simulink model "GridN4"  (R2021a)
settings: Solver=FixedStepAuto  StartTime=0.0  StopTime=0.2  FixedStep=0.2  RelTol=1e-3
libraries: spsDistributedParametersLineLib x13, spsThreePhaseSeriesRLCLoadLib x6, spsThreePhaseVIMeasurementLib x2, spsGroundLib x1, spsThreePhaseSourceLib x1, spsSeriesRLCBranchLib x1, spspowerguiLib x1
settings Model: Creator=miair  LastModifiedBy=Admin
settings SolverCC: AlgebraicLoopSolver=TrustRegion
settings DataIOCC: ReturnWorkspaceOutputs=off
settings DebuggingCC: SFMachineParentedDataDiag=warning  ArithmeticOperatorsInVariantConditions=warning
settings SFSimCC: SimUseLocalCustomCode=off  CustomCodeUndefinedFunction=UseInterfaceOnly
settings RTWCC: RTWUseLocalCustomCode=off
settings CodeAppCC: StateflowObjectComments=on
settings SimscapeCC: SimscapeNormalizeSystem=off

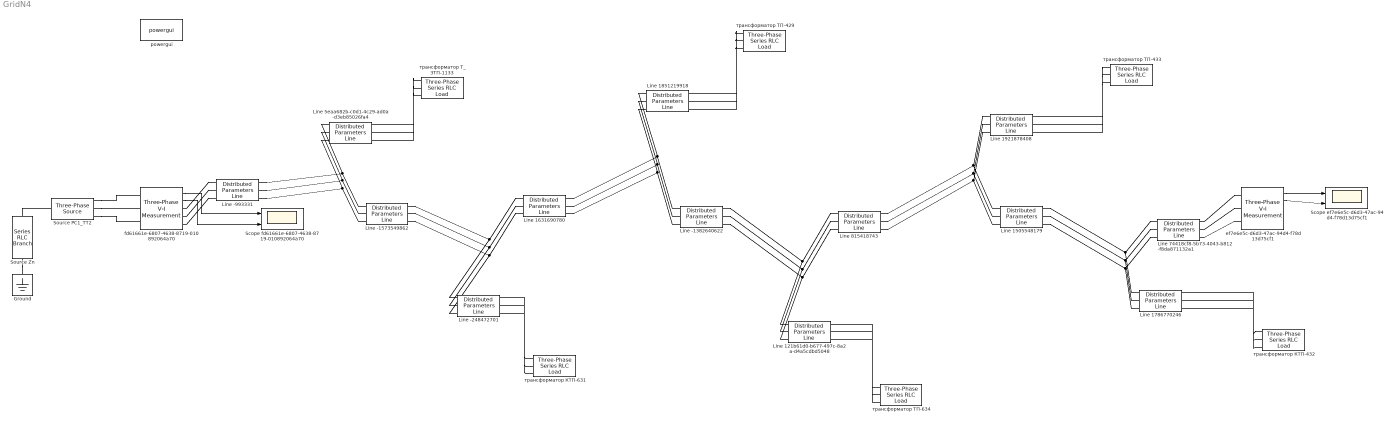
== system GridN4 ==
  Ground : spsGroundLib/Ground  LConnTagsString=a
  Line -1382640622 : spsDistributedParametersLineLib/Distributed Parameters Line  Description=|  Phases=3  Length=1.4772  Frequency=50  Resistance=[0.646656091154803 0.0486237908083191 0.0486712220507153;0.0486237908083191 0.646561225344642 0.0486237934466192;0.0486712220507153 0.0486237934466192 0.646656091154803]  Inductance=[0.00282448912315926 0.00133270803418135 0.00132951476746136;0.00133270803418135 0.00282479813276775 0.00133799988507366;0.00132951476746136 0.00133799988507366 0.00282448912315926]  Capacitance=[7.89543174552926e-09 -1.85986777702161e-09 -1.7901190036642e-09;-1.85986777702161e-09 7.82540023894543e-09 -1.8957321828871e-09;-1.7901190036642e-09 -1.8957321828871e-09 7.91264394645417e-09]  x1=[85.8857792377858 6510.87905206758 6510.37512083704;314.159265358979 314.159265358979 314.159265358979;0.297795361599447 -0.904054654199639 -2.47497799182329]  x2=[85.9647541006012 6498.88512116897 6498.39920566151;314.159265358979 314.159265358979 314.159265358979;0.29836012891069 -0.904731827544364 -2.47564826583381]  x3=[0.104217124772641 6.72029956175141 6.82412580592181;314.159265358979 314.159265358979 314.159265358979;0.111414320617144 -0.3562443922381 -1.93698471339142]  x4=[0.0514466308166242 27.5442395111353 27.6704588799536;314.159265358979 314.159265358979 314.159265358979;0.679987114816006 -1.03294818731528 -2.60316864161815]  x5=7.07796349106919e-06  V1=ones(3,3)  V2=ones(3,3)  I1=ones(3,3)  I2=ones(3,3)  nHarmo=1  Measurements=None  Decoupling=off  VsMag0=0  VrMag0=0  VsAngle0=0  VrAngle0=0  IsMag0=0  IrMag0=0  IsAngle0=0  IrAngle0=0
      | Line connected to devices: [Опора-4/1_Л-8-10кВ_Воробьево
      | Опора-2/44_Л-8-10кВ_Воробьево, Опора-2/67_Л-8-10кВ_Воробьево]
      settings: SourceProductBaseCode=PS
  Line -1573549862 : spsDistributedParametersLineLib/Distributed Parameters Line  Description=|  Phases=3  Length=0.98898  Frequency=50  Resistance=[0.646656091154803 0.0486237908083191 0.0486712220507153;0.0486237908083191 0.646561225344642 0.0486237934466192;0.0486712220507153 0.0486237934466192 0.646656091154803]  Inductance=[0.00282448912315926 0.00133270803418135 0.00132951476746136;0.00133270803418135 0.00282479813276775 0.00133799988507366;0.00132951476746136 0.00133799988507366 0.00282448912315926]  Capacitance=[7.89543174552926e-09 -1.85986777702161e-09 -1.7901190036642e-09;-1.85986777702161e-09 7.82540023894543e-09 -1.8957321828871e-09;-1.7901190036642e-09 -1.8957321828871e-09 7.91264394645417e-09]  x1=[85.6677259618718 6543.90351776437 6543.34962523968;314.159265358979 314.159265358979 314.159265358979;0.296971250306257 -0.901609957237111 -2.47255157035452]  x2=[85.7598900271541 6529.94544416512 6529.41271684245;314.159265358979 314.159265358979 314.159265358979;0.297631180119223 -0.902394975430767 -2.473328653112]  x3=[0.127076602259962 6.46782645683811 6.42234305042791;314.159265358979 314.159265358979 314.159265358979;0.0294613778206171 1.00930239141356 -0.579244928461238]  x4=[0.0432092930617411 35.9185691148936 36.0457502607365;314.159265358979 314.159265358979 314.159265358979;1.18518823340833 -1.07311367571862 -2.64327629161882]  x5=4.73867068331817e-06  V1=ones(3,3)  V2=ones(3,3)  I1=ones(3,3)  I2=ones(3,3)  nHarmo=1  Measurements=None  Decoupling=off  VsMag0=0  VrMag0=0  VsAngle0=0  VrAngle0=0  IsMag0=0  IrMag0=0  IsAngle0=0  IrAngle0=0
      | Line connected to devices: [СШ ЗТП-1133, Опора-3/1_Л-8-10кВ_Воробьево
      | Опора-2/16_Л-8-10кВ_Воробьево]
      settings: SourceProductBaseCode=PS
  Line -248472701 : spsDistributedParametersLineLib/Distributed Parameters Line  Description=|  Phases=3  Length=0.18015  Frequency=50  Resistance=[0.646656091154803 0.0486237908083191 0.0486712220507153;0.0486237908083191 0.646561225344642 0.0486237934466192;0.0486712220507153 0.0486237934466192 0.646656091154803]  Inductance=[0.00282448912315926 0.00133270803418135 0.00132951476746136;0.00133270803418135 0.00282479813276775 0.00133799988507366;0.00132951476746136 0.00133799988507366 0.00282448912315926]  Capacitance=[7.89543174552926e-09 -1.85986777702161e-09 -1.7901190036642e-09;-1.85986777702161e-09 7.82540023894543e-09 -1.8957321828871e-09;-1.7901190036642e-09 -1.8957321828871e-09 7.91264394645417e-09]  x1=[85.7598900271543 6529.94544416512 6529.41271684245;314.159265358979 314.159265358979 314.159265358979;0.298848700228514 -0.901427735668235 -2.4723604926057]  x2=[85.763454791984 6529.39738401349 6528.86547736649;314.159265358979 314.159265358979 314.159265358979;0.298874766091125 -0.901458260199312 -2.47239070103001]  x3=[0.0855260327133963 12.6404163140629 12.764989480605;314.159265358979 314.159265358979 314.159265358979;0.215972029306597 -0.796300987449647 -2.3683442154795]  x4=[0.0651073125741442 20.6999331634113 20.8266702112825;314.159265358979 314.159265358979 314.159265358979;0.407523776195381 -0.965746971947712 -2.53623983661103]  x5=8.63183809176898e-07  V1=ones(3,3)  V2=ones(3,3)  I1=ones(3,3)  I2=ones(3,3)  nHarmo=1  Measurements=None  Decoupling=off  VsMag0=0  VrMag0=0  VsAngle0=0  VrAngle0=0  IsMag0=0  IrMag0=0  IsAngle0=0  IrAngle0=0
      | Line connected to devices: [Опора-3/1_Л-8-10кВ_Воробьево
      | Опора-2/16_Л-8-10кВ_Воробьево, трансформатор КТП-631]
      settings: SourceProductBaseCode=PS
  Line -993331 : spsDistributedParametersLineLib/Distributed Parameters Line  Description=Line connected to devices: [ВВ Ячейка_Л-8-10кВ_Воробьево, СШ ЗТП-1133]  Phases=3  Length=0.892  Frequency=50  Resistance=[0.646656091154803 0.0486237908083191 0.0486712220507153;0.0486237908083191 0.646561225344642 0.0486237934466192;0.0486712220507153 0.0486237934466192 0.646656091154803]  Inductance=[0.00282448912315926 0.00133270803418135 0.00132951476746136;0.00133270803418135 0.00282479813276775 0.00133799988507366;0.00132951476746136 0.00133799988507366 0.00282448912315926]  Capacitance=[7.89543174552926e-09 -1.85986777702161e-09 -1.7901190036642e-09;-1.85986777702161e-09 7.82540023894543e-09 -1.8957321828871e-09;-1.7901190036642e-09 -1.8957321828871e-09 7.91264394645417e-09]  x1=[85.5017510654121 6569.24560507323 6568.65333179846;314.159265358979 314.159265358979 314.159265358979;0.295910641359064 -0.900082774080867 -2.47103868556443]  x2=[85.667725961872 6543.90351776437 6543.34962523968;314.159265358979 314.159265358979 314.159265358979;0.297117232898643 -0.901493983655308 -2.47243548637407]  x3=[0.183284202527258 24.4320765018378 24.3241695261716;314.159265358979 314.159265358979 314.159265358979;-0.0762727108476125 1.71053738269408 0.137523096986334]  x4=[0.0699142754394648 55.8037793342115 55.9323018365664;314.159265358979 314.159265358979 314.159265358979;2.17390443481334 -1.12439915077923 -2.69462173279304]  x5=4.27399365964914e-06  V1=ones(3,3)  V2=ones(3,3)  I1=ones(3,3)  I2=ones(3,3)  nHarmo=1  Measurements=None  Decoupling=off  VsMag0=0  VrMag0=0  VsAngle0=0  VrAngle0=0  IsMag0=0  IrMag0=0  IsAngle0=0  IrAngle0=0
      settings: SourceProductBaseCode=PS
  Line 121b61d0-b677-497c-8a2a-d4a5cdbd5048 : spsDistributedParametersLineLib/Distributed Parameters Line  Description=Line connected to devices: [Опора-2/67_Л-8-10кВ_Воробьево, трансформатор ТП-634]  Phases=3  Length=0.01635  Frequency=50  Resistance=[0.646656091154803 0.0486237908083191 0.0486712220507153;0.0486237908083191 0.646561225344642 0.0486237934466192;0.0486712220507153 0.0486237934466192 0.646656091154803]  Inductance=[0.00282448912315926 0.00133270803418135 0.00132951476746136;0.00133270803418135 0.00282479813276775 0.00133799988507366;0.00132951476746136 0.00133799988507366 0.00282448912315926]  Capacitance=[7.89543174552926e-09 -1.85986777702161e-09 -1.7901190036642e-09;-1.85986777702161e-09 7.82540023894543e-09 -1.8957321828871e-09;-1.7901190036642e-09 -1.8957321828871e-09 7.91264394645417e-09]  x1=[85.9647541006012 6498.88512116897 6498.39920566151;314.159265358979 314.159265358979 314.159265358979;0.300559125302584 -0.902984869336713 -2.47389964464565]  x2=[85.9650422946656 6498.84085463915 6498.3550050936;314.159265358979 314.159265358979 314.159265358979;0.300561215685984 -0.902987343814113 -2.47390209345756]  x3=[0.0845031718933416 12.9941072057686 13.1185063261115;314.159265358979 314.159265358979 314.159265358979;0.225790596837781 -0.81181384254389 -2.38366283032811]  x4=[0.0663567082392332 20.1717718047634 20.2980663663425;314.159265358979 314.159265358979 314.159265358979;0.395804226320378 -0.961685203465561 -2.53219107175892]  x5=7.83405788511923e-08  V1=ones(3,3)  V2=ones(3,3)  I1=ones(3,3)  I2=ones(3,3)  nHarmo=1  Measurements=None  Decoupling=off  VsMag0=0  VrMag0=0  VsAngle0=0  VrAngle0=0  IsMag0=0  IrMag0=0  IsAngle0=0  IrAngle0=0
      settings: SourceProductBaseCode=PS
  Line 1505548179 : spsDistributedParametersLineLib/Distributed Parameters Line  Description=|  Phases=3  Length=0.64126  Frequency=50  Resistance=[0.646656091154803 0.0486237908083191 0.0486712220507153;0.0486237908083191 0.646561225344642 0.0486237934466192;0.0486712220507153 0.0486237934466192 0.646656091154803]  Inductance=[0.00282448912315926 0.00133270803418135 0.00132951476746136;0.00133270803418135 0.00282479813276775 0.00133799988507366;0.00132951476746136 0.00133799988507366 0.00282448912315926]  Capacitance=[7.89543174552926e-09 -1.85986777702161e-09 -1.7901190036642e-09;-1.85986777702161e-09 7.82540023894543e-09 -1.8957321828871e-09;-1.7901190036642e-09 -1.8957321828871e-09 7.91264394645417e-09]  x1=[85.9782141140988 6496.83974420136 6496.35689426354;314.159265358979 314.159265358979 314.159265358979;0.299714694293971 -0.903847773979785 -2.47476208082445]  x2=[85.9863685586919 6495.60045471061 6495.11946118362;314.159265358979 314.159265358979 314.159265358979;0.299772995272737 -0.903917843201306 -2.47483143467166]  x3=[0.0817935347341075 13.9726348442168 14.0973824230101;314.159265358979 314.159265358979 314.159265358979;0.243299003310729 -0.844416769677226 -2.4159125997663]  x4=[0.0687945310174185 19.1108172128254 19.2367683619024;314.159265358979 314.159265358979 314.159265358979;0.365811974240705 -0.948012410065521 -2.51860256931505]  x5=3.07257979168902e-06  V1=ones(3,3)  V2=ones(3,3)  I1=ones(3,3)  I2=ones(3,3)  nHarmo=1  Measurements=None  Decoupling=off  VsMag0=0  VrMag0=0  VsAngle0=0  VrAngle0=0  IsMag0=0  IrMag0=0  IsAngle0=0  IrAngle0=0
      | Line connected to devices: [Опора-5/11_Л-8-10кВ_Воробьево, Опора-5/22_Л-8-10кВ_Воробьево
      | Опора-6/1_Л-8-10кВ_Воробьево]
      settings: SourceProductBaseCode=PS
  Line 1631690780 : spsDistributedParametersLineLib/Distributed Parameters Line  Description=|  Phases=3  Length=1.7207  Frequency=50  Resistance=[0.646656091154803 0.0486237908083191 0.0486712220507153;0.0486237908083191 0.646561225344642 0.0486237934466192;0.0486712220507153 0.0486237934466192 0.646656091154803]  Inductance=[0.00282448912315926 0.00133270803418135 0.00132951476746136;0.00133270803418135 0.00282479813276775 0.00133799988507366;0.00132951476746136 0.00133799988507366 0.00282448912315926]  Capacitance=[7.89543174552926e-09 -1.85986777702161e-09 -1.7901190036642e-09;-1.85986777702161e-09 7.82540023894543e-09 -1.8957321828871e-09;-1.7901190036642e-09 -1.8957321828871e-09 7.91264394645417e-09]  x1=[85.7598900271543 6529.94544416512 6529.41271684245;314.159265358979 314.159265358979 314.159265358979;0.296529732578495 -0.903270003160994 -2.47420451380666]  x2=[85.885779237786 6510.87905206758 6510.37512083704;314.159265358979 314.159265358979 314.159265358979;0.297428824568657 -0.904345843797177 -2.4752694586127]  x3=[0.115392677686701 5.11554930731978 5.15645833165549;314.159265358979 314.159265358979 314.159265358979;0.0654720110181994 0.300032187240473 -1.29342773701317]  x4=[0.0459043551859802 31.654468125409 31.780923150932;314.159265358979 314.159265358979 314.159265358979;0.906579123862255 -1.05632172807641 -2.62649842032608]  x5=8.24468709659e-06  V1=ones(3,3)  V2=ones(3,3)  I1=ones(3,3)  I2=ones(3,3)  nHarmo=1  Measurements=None  Decoupling=off  VsMag0=0  VrMag0=0  VsAngle0=0  VrAngle0=0  IsMag0=0  IrMag0=0  IsAngle0=0  IrAngle0=0
      | Line connected to devices: [Опора-3/1_Л-8-10кВ_Воробьево
      | Опора-2/16_Л-8-10кВ_Воробьево, Опора-4/1_Л-8-10кВ_Воробьево
      | Опора-2/44_Л-8-10кВ_Воробьево]
      settings: SourceProductBaseCode=PS
  Line 1786770246 : spsDistributedParametersLineLib/Distributed Parameters Line  Description=|  Phases=3  Length=0.1272  Frequency=50  Resistance=[0.646656091154803 0.0486237908083191 0.0486712220507153;0.0486237908083191 0.646561225344642 0.0486237934466192;0.0486712220507153 0.0486237934466192 0.646656091154803]  Inductance=[0.00282448912315926 0.00133270803418135 0.00132951476746136;0.00133270803418135 0.00282479813276775 0.00133799988507366;0.00132951476746136 0.00133799988507366 0.00282448912315926]  Capacitance=[7.89543174552926e-09 -1.85986777702161e-09 -1.7901190036642e-09;-1.85986777702161e-09 7.82540023894543e-09 -1.8957321828871e-09;-1.7901190036642e-09 -1.8957321828871e-09 7.91264394645417e-09]  x1=[85.986368558692 6495.60045471061 6495.11946118362;314.159265358979 314.159265358979 314.159265358979;0.300546802361227 -0.903303104291613 -2.47421611057405]  x2=[85.987974719349 6495.35409079703 6494.87346443576;314.159265358979 314.159265358979 314.159265358979;0.300558422703274 -0.903316900029618 -2.47422976347415]  x3=[0.0818157857085095 13.9789572696683 14.1038243366368;314.159265358979 314.159265358979 314.159265358979;0.245124873008095 -0.842873708994508 -2.41436845595092]  x4=[0.0688122190292833 19.1210807902262 19.2471828808458;314.159265358979 314.159265358979 314.159265358979;0.366258973448979 -0.947612594243962 -2.51820244936986]  x5=6.09475329044138e-07  V1=ones(3,3)  V2=ones(3,3)  I1=ones(3,3)  I2=ones(3,3)  nHarmo=1  Measurements=None  Decoupling=off  VsMag0=0  VrMag0=0  VsAngle0=0  VrAngle0=0  IsMag0=0  IrMag0=0  IsAngle0=0  IrAngle0=0
      | Line connected to devices: [Опора-5/22_Л-8-10кВ_Воробьево
      | Опора-6/1_Л-8-10кВ_Воробьево, трансформатор КТП-432]
      settings: SourceProductBaseCode=PS
  Line 1851219918 : spsDistributedParametersLineLib/Distributed Parameters Line  Description=|  Phases=3  Length=0.32675  Frequency=50  Resistance=[0.80718830189013 0.0486237908083191 0.0486712220507153;0.0486237908083191 0.807093436079969 0.0486237934466192;0.0486712220507153 0.0486237934466192 0.80718830189013]  Inductance=[0.00279786707424938 0.00133270803418135 0.00132951476746136;0.00133270803418135 0.00279817608385787 0.00133799988507366;0.00132951476746136 0.00133799988507366 0.00279786707424938]  Capacitance=[7.73340098830622e-09 -1.79942827973291e-09 -1.73218055098733e-09;-1.79942827973291e-09 7.66505189233746e-09 -1.83375898618858e-09;-1.73218055098733e-09 -1.83375898618858e-09 7.749673531177e-09]  x1=[35.0955610217797 6510.93626861035 6510.47784355858;314.159265358979 314.159265358979 314.159265358979;0.364048571301998 -0.906982844271675 -2.4778653146309]  x2=[35.1090749306274 6509.76050560653 6509.30346363258;314.159265358979 314.159265358979 314.159265358979;0.364282153710788 -0.907025083589128 -2.47790699244812]  x3=[0.053546825388311 12.6323991504187 12.7556347743014;314.159265358979 314.159265358979 314.159265358979;0.121698475744269 -0.804373284979287 -2.37631014198273]  x4=[0.0157903814772497 20.5120745317561 20.6371829254422;314.159265358979 314.159265358979 314.159265358979;1.31388432987898 -0.970449254624203 -2.54091211842884]  x5=1.55396258303596e-06  V1=ones(3,3)  V2=ones(3,3)  I1=ones(3,3)  I2=ones(3,3)  nHarmo=1  Measurements=None  Decoupling=off  VsMag0=0  VrMag0=0  VsAngle0=0  VrAngle0=0  IsMag0=0  IrMag0=0  IsAngle0=0  IrAngle0=0
      | Line connected to devices: [Опора-4/1_Л-8-10кВ_Воробьево
      | Опора-2/44_Л-8-10кВ_Воробьево, трансформатор ТП-429]
      settings: SourceProductBaseCode=PS
  Line 1921878408 : spsDistributedParametersLineLib/Distributed Parameters Line  Description=Line connected to devices: [Опора-5/11_Л-8-10кВ_Воробьево, трансформатор ТП-433]  Phases=3  Length=0.4618  Frequency=50  Resistance=[0.646656091154803 0.0486237908083191 0.0486712220507153;0.0486237908083191 0.646561225344642 0.0486237934466192;0.0486712220507153 0.0486237934466192 0.646656091154803]  Inductance=[0.00282448912315926 0.00133270803418135 0.00132951476746136;0.00133270803418135 0.00282479813276775 0.00133799988507366;0.00132951476746136 0.00133799988507366 0.00282448912315926]  Capacitance=[7.89543174552926e-09 -1.85986777702161e-09 -1.7901190036642e-09;-1.85986777702161e-09 7.82540023894543e-09 -1.8957321828871e-09;-1.7901190036642e-09 -1.8957321828871e-09 7.91264394645417e-09]  x1=[85.9782141140988 6496.83974420136 6496.35689426354;314.159265358979 314.159265358979 314.159265358979;0.299984832838304 -0.903633166648475 -2.47454726920216]  x2=[85.9887456902377 6495.22639796506 6494.74595450459;314.159265358979 314.159265358979 314.159265358979;0.300060905853593 -0.903723616816745 -2.4746367847328]  x3=[0.0872953522522821 11.9773450357035 12.1008086534499;314.159265358979 314.159265358979 314.159265358979;0.205888555546858 -0.776499548323462 -2.34881902331988]  x4=[0.0639360316201987 21.2204566545086 21.3466472540646;314.159265358979 314.159265358979 314.159265358979;0.427890764596808 -0.975760358930525 -2.54619369646504]  x5=2.21270209868383e-06  V1=ones(3,3)  V2=ones(3,3)  I1=ones(3,3)  I2=ones(3,3)  nHarmo=1  Measurements=None  Decoupling=off  VsMag0=0  VrMag0=0  VsAngle0=0  VrAngle0=0  IsMag0=0  IrMag0=0  IsAngle0=0  IrAngle0=0
      settings: SourceProductBaseCode=PS
  Line 5eaa682b-c0d1-4c29-ad0a-d3eb85026fa4 : spsDistributedParametersLineLib/Distributed Parameters Line  Description=Line connected to devices: [СШ ЗТП-1133, трансформатор Т_ЗТП-1133]  Phases=3  Length=0.005  Frequency=50  Resistance=[0.476003738225748 0.351747138225748 0.351747138225748;0.351747138225748 0.476003738225748 0.351747138225748;0.351747138225748 0.351747138225748 0.476003738225748]  Inductance=[0.000705954362986426 0.000459934243504405 0.000459934243504405;0.000459934243504405 0.000705954362986426 0.000459934243504405;0.000459934243504405 0.000459934243504405 0.000705954362986426]  Capacitance=[5.7561313269996e-07 -1.37543883484145e-07 -1.37543912800485e-07;-1.37543883484145e-07 5.75613027339387e-07 -1.37543875208088e-07;-1.37543912800485e-07 -1.37543875208088e-07 5.75613005057695e-07]  x1=[0.54450777408875 6544.57939789872 6544.6295286263;314.159265358979 314.159265358979 314.159265358979;0.714768245227439 -0.81880232697569 -2.38958538171649]  x2=[0.544507775115402 6544.56517823051 6544.61530884916;314.159265358979 314.159265358979 314.159265358979;0.714768249538482 -0.818802856525843 -2.38958591126664]  x3=[0.00740285087456037 333.407343244233 333.409869872674;314.159265358979 314.159265358979 314.159265358979;0.714787417474713 -0.800088267408842 -2.37087132057921]  x4=[0.00740226634003595 371.409022497912 371.411840212342;314.159265358979 314.159265358979 314.159265358979;0.71471415547024 -0.835621662804389 -2.40640471880579]  x5=1.10521588109605e-07  V1=ones(3,3)  V2=ones(3,3)  I1=ones(3,3)  I2=ones(3,3)  nHarmo=1  Measurements=None  Decoupling=off  VsMag0=0  VrMag0=0  VsAngle0=0  VrAngle0=0  IsMag0=0  IrMag0=0  IsAngle0=0  IrAngle0=0
      settings: SourceProductBaseCode=PS
  Line 74418cf8-5b73-4043-b812-f8da871132a1 : spsDistributedParametersLineLib/Distributed Parameters Line  Description=|  Phases=3  Length=0.075191  Frequency=50  Resistance=[0.646656091154803 0.0486237908083191 0.0486712220507153;0.0486237908083191 0.646561225344642 0.0486237934466192;0.0486712220507153 0.0486237934466192 0.646656091154803]  Inductance=[0.00282448912315926 0.00133270803418135 0.00132951476746136;0.00133270803418135 0.00282479813276775 0.00133799988507366;0.00132951476746136 0.00133799988507366 0.00282448912315926]  Capacitance=[7.89543174552926e-09 -1.85986777702161e-09 -1.7901190036642e-09;-1.85986777702161e-09 7.82540023894543e-09 -1.8957321828871e-09;-1.7901190036642e-09 -1.8957321828871e-09 7.91264394645417e-09]  x1=[85.986368558692 6495.60045471061 6495.11946118362;314.159265358979 314.159265358979 314.159265358979;0.30062509075726 -0.90324090930279 -2.47415385638001]  x2=[85.9863691094628 6495.6004809694 6495.11948749048;314.159265358979 314.159265358979 314.159265358979;0.30062508799497 -0.903240914446174 -2.47415386156691]  x3=[0.0751781366141678 16.5291718714337 16.6548812296208;314.159265358979 314.159265358979 314.159265358979;0.300511905231519 -0.903330829071536 -2.47424386176377]  x4=[0.0751781366044267 16.5291718713753 16.6548812296373;314.159265358979 314.159265358979 314.159265358979;0.300625088102045 -0.903240914444271 -2.47415386156555]  x5=3.60275624733945e-07  V1=ones(3,3)  V2=ones(3,3)  I1=ones(3,3)  I2=ones(3,3)  nHarmo=1  Measurements=None  Decoupling=off  VsMag0=0  VrMag0=0  VsAngle0=0  VrAngle0=0  IsMag0=0  IrMag0=0  IsAngle0=0  IrAngle0=0
      | Line connected to devices: [Опора-5/22_Л-8-10кВ_Воробьево
      | Опора-6/1_Л-8-10кВ_Воробьево, ВВ РВА-9-10кВ]
      settings: SourceProductBaseCode=PS
  Line 815418743 : spsDistributedParametersLineLib/Distributed Parameters Line  Description=Line connected to devices: [Опора-2/67_Л-8-10кВ_Воробьево, Опора-5/11_Л-8-10кВ_Воробьево]  Phases=3  Length=0.37741  Frequency=50  Resistance=[0.646656091154803 0.0486237908083191 0.0486712220507153;0.0486237908083191 0.646561225344642 0.0486237934466192;0.0486712220507153 0.0486237934466192 0.646656091154803]  Inductance=[0.00282448912315926 0.00133270803418135 0.00132951476746136;0.00133270803418135 0.00282479813276775 0.00133799988507366;0.00132951476746136 0.00133799988507366 0.00282448912315926]  Capacitance=[7.89543174552926e-09 -1.85986777702161e-09 -1.7901190036642e-09;-1.85986777702161e-09 7.82540023894543e-09 -1.8957321828871e-09;-1.7901190036642e-09 -1.8957321828871e-09 7.91264394645417e-09]  x1=[85.9647541006012 6498.88512116897 6498.39920566151;314.159265358979 314.159265358979 314.159265358979;0.300015626902847 -0.903416643119411 -2.47433182944641]  x2=[85.9782141140989 6496.83974420136 6496.35689426354;314.159265358979 314.159265358979 314.159265358979;0.300111863885648 -0.903532248824507 -2.47444625531157]  x3=[0.0942961521230071 9.6032487634775 9.72315536893301;314.159265358979 314.159265358979 314.159265358979;0.163257520349026 -0.657036880008762 -2.23127062356536]  x4=[0.0583189637097579 23.861361569197 23.9877628443537;314.159265358979 314.159265358979 314.159265358979;0.52165372229803 -1.00212752075027 -2.5724370096926]  x5=1.80834971646657e-06  V1=ones(3,3)  V2=ones(3,3)  I1=ones(3,3)  I2=ones(3,3)  nHarmo=1  Measurements=None  Decoupling=off  VsMag0=0  VrMag0=0  VsAngle0=0  VrAngle0=0  IsMag0=0  IrMag0=0  IsAngle0=0  IrAngle0=0
      settings: SourceProductBaseCode=PS
  Scope ef7e6e5c-d6d3-47ac-94d4-f78d13d75cf1 : Scope  NumInputPorts=2
  Scope fd61661e-6807-4638-8719-010892064a70 : Scope  NumInputPorts=2
  Source PC1_TT2 : spsThreePhaseSourceLib/Three-Phase Source  InternalConnection=Yn  VoltagePhases=off  Voltage=10000  PhaseAngle=0  Voltage_phases=[25e3 25e3 25e3]/sqrt(3)  PhaseAngles_phases=[0 -120 +120]  Frequency=50  NonIdealSource=on  SpecifyImpedance=off  Resistance=0.14  Inductance=0.0031831  ShortCircuitLevel=100e6  BaseVoltage=25e3  XRratio=7  BusType=swing  Pref=10e3  Qref=0  Prefabc=[10e3, 10e3, 10e3]  Qrefabc=[0, 0, 0]  Qmin=-inf  Qmax=inf
  Source Zn : spsSeriesRLCBranchLib/Series RLC Branch  LConnTagsString=__new0  RConnTagsString=__new0  BranchType=RL  Resistance=0.001  Inductance=3.1831e-06  SetiL0=off  InitialCurrent=0  Capacitance=0  Setx0=off  InitialVoltage=0  Measurements=None
  ef7e6e5c-d6d3-47ac-94d4-f78d13d75cf1 : spsThreePhaseVIMeasurementLib/Three-Phase V-I Measurement  VoltageMeasurement=phase-to-ground  SetLabelV=off  LabelV=Vabc  Vpu=off  VpuLL=off  CurrentMeasurement=yes  SetLabelI=off  LabelI=Iabc  Ipu=off  Pbase=100e6  Vbase=500e3  OutputType=Complex  PhasorSimulation=on  PSBequivalent=0
  fd61661e-6807-4638-8719-010892064a70 : spsThreePhaseVIMeasurementLib/Three-Phase V-I Measurement  VoltageMeasurement=phase-to-ground  SetLabelV=off  LabelV=Vabc  Vpu=off  VpuLL=off  CurrentMeasurement=yes  SetLabelI=off  LabelI=Iabc  Ipu=off  Pbase=100e6  Vbase=500e3  OutputType=Complex  PhasorSimulation=on  PSBequivalent=0
  powergui : spspowerguiLib/powergui  Priority=1  SimulationMode=Phasor  SampleTime=50e-6  frequency=50  Iterations=50  frequencyindice=50  Pbase=100e6  ErrMax=1e-4  UnitsV=kV  UnitsW=MW  buscounter=0  FunctionMessages=off  echomessages=off  EnableUseOfTLC=off  CurrentSourceSwitches=off  DisableSnubberDevices=off  DisableRonSwitches=off  DisableVfSwitches=off  DisplayEquations=off  AutomaticDiscreteSolvers=off  SolverType=Tustin/Backward Euler (TBE)  Interpol=off  ExternalGateDelay=off  methode=off  Ts=10  x0status=blocks  SPID=off  SwTol=0  HookPort=off  NonlinearTolerance=1e-4  nMaxIteration=100  ContinueOnMaxIteration=off  RestoreLinks=warning  ResistiveCurrentMeasurement=off  Frange=[0:2:500]  Ylog=off  Xlog=on  ShowGrid=off  save=off  variable=ZData  structure=0  ZoomFFT=off  StartTime=0.0  cycles=1  DisplayStyle=1  fundamental=60  FreqAxis=off  MaxFrequency=1000  frequencyindicesteady=1  RmsSteady=1  display=off
  трансформатор КТП-432 : spsThreePhaseSeriesRLCLoadLib/Three-Phase Series RLC Load  Description=Device type: [LOAD], in DispatcherName: [трансформатор КТП-432]  LConnTagsString=A|B|C  Configuration=Delta  NominalVoltage=10500  Vabc=[1e3 1e3 1e3]  Vabcp=[1e3 1e3 1e3]  NominalFrequency=50  UnbalancedPower=off  ActivePower=43700  InductivePower=14363.495  CapacitivePower=0  Pabc=[10e3 9e3 11e3]  QLabc=[100 90 110]  QCabc=[100 90 110]  Pabcp=[10e3 9e3 11e3]  QLabcp=[100 90 110]  QCabcp=[100 90 110]  Measurements=None  LoadType=constant Z
  трансформатор КТП-631 : spsThreePhaseSeriesRLCLoadLib/Three-Phase Series RLC Load  Description=Device type: [LOAD], in DispatcherName: [трансформатор КТП-631]  LConnTagsString=A|B|C  Configuration=Delta  NominalVoltage=10500  Vabc=[1e3 1e3 1e3]  Vabcp=[1e3 1e3 1e3]  NominalFrequency=50  UnbalancedPower=off  ActivePower=68281.25  InductivePower=22442.962  CapacitivePower=0  Pabc=[10e3 9e3 11e3]  QLabc=[100 90 110]  QCabc=[100 90 110]  Pabcp=[10e3 9e3 11e3]  QLabcp=[100 90 110]  QCabcp=[100 90 110]  Measurements=None  LoadType=constant Z
  трансформатор Т_ЗТП-1133 : spsThreePhaseSeriesRLCLoadLib/Three-Phase Series RLC Load  Description=Device type: [LOAD], in DispatcherName: [трансформатор Т_ЗТП-1133]  LConnTagsString=A|B|C  Configuration=Delta  NominalVoltage=10500  Vabc=[1e3 1e3 1e3]  Vabcp=[1e3 1e3 1e3]  NominalFrequency=50  UnbalancedPower=off  ActivePower=320150  InductivePower=105228.216  CapacitivePower=0  Pabc=[10e3 9e3 11e3]  QLabc=[100 90 110]  QCabc=[100 90 110]  Pabcp=[10e3 9e3 11e3]  QLabcp=[100 90 110]  QCabcp=[100 90 110]  Measurements=None  LoadType=constant Z
  трансформатор ТП-429 : spsThreePhaseSeriesRLCLoadLib/Three-Phase Series RLC Load  Description=Device type: [LOAD], in DispatcherName: [трансформатор ТП-429]  LConnTagsString=A|B|C  Configuration=Delta  NominalVoltage=10500  Vabc=[1e3 1e3 1e3]  Vabcp=[1e3 1e3 1e3]  NominalFrequency=50  UnbalancedPower=off  ActivePower=66975  InductivePower=22013.618  CapacitivePower=0  Pabc=[10e3 9e3 11e3]  QLabc=[100 90 110]  QCabc=[100 90 110]  Pabcp=[10e3 9e3 11e3]  QLabcp=[100 90 110]  QCabcp=[100 90 110]  Measurements=None  LoadType=constant Z
  трансформатор ТП-433 : spsThreePhaseSeriesRLCLoadLib/Three-Phase Series RLC Load  Description=Device type: [LOAD], in DispatcherName: [трансформатор ТП-433]  LConnTagsString=A|B|C  Configuration=Delta  NominalVoltage=10500  Vabc=[1e3 1e3 1e3]  Vabcp=[1e3 1e3 1e3]  NominalFrequency=50  UnbalancedPower=off  ActivePower=78850  InductivePower=25916.742  CapacitivePower=0  Pabc=[10e3 9e3 11e3]  QLabc=[100 90 110]  QCabc=[100 90 110]  Pabcp=[10e3 9e3 11e3]  QLabcp=[100 90 110]  QCabcp=[100 90 110]  Measurements=None  LoadType=constant Z
  трансформатор ТП-634 : spsThreePhaseSeriesRLCLoadLib/Three-Phase Series RLC Load  Description=Device type: [LOAD], in DispatcherName: [трансформатор ТП-634]  LConnTagsString=A|B|C  Configuration=Delta  NominalVoltage=10500  Vabc=[1e3 1e3 1e3]  Vabcp=[1e3 1e3 1e3]  NominalFrequency=50  UnbalancedPower=off  ActivePower=61037.5  InductivePower=20062.056  CapacitivePower=0  Pabc=[10e3 9e3 11e3]  QLabc=[100 90 110]  QCabc=[100 90 110]  Pabcp=[10e3 9e3 11e3]  QLabcp=[100 90 110]  QCabcp=[100 90 110]  Measurements=None  LoadType=constant Z
  wires:
  fd61661e-6807-4638-8719-010892064a70/1 -> Scope fd61661e-6807-4638-8719-010892064a70/1
  fd61661e-6807-4638-8719-010892064a70/2 -> Scope fd61661e-6807-4638-8719-010892064a70/2
  ef7e6e5c-d6d3-47ac-94d4-f78d13d75cf1/1 -> Scope ef7e6e5c-d6d3-47ac-94d4-f78d13d75cf1/1
  ef7e6e5c-d6d3-47ac-94d4-f78d13d75cf1/2 -> Scope ef7e6e5c-d6d3-47ac-94d4-f78d13d75cf1/2
  connections:
  Source Zn/LConn1 -- Ground/LConn1
  Source Zn/RConn1 -- Source PC1_TT2/LConn1
  Line 815418743/LConn1 -- Line -1382640622/RConn1 -- Line 121b61d0-b677-497c-8a2a-d4a5cdbd5048/LConn1
  Line 815418743/LConn2 -- Line -1382640622/RConn2 -- Line 121b61d0-b677-497c-8a2a-d4a5cdbd5048/LConn2
  Line 815418743/LConn3 -- Line -1382640622/RConn3 -- Line 121b61d0-b677-497c-8a2a-d4a5cdbd5048/LConn3
  Line 1631690780/LConn1 -- Line -1573549862/RConn1 -- Line -248472701/LConn1
  Line 1631690780/LConn2 -- Line -1573549862/RConn2 -- Line -248472701/LConn2
  Line 1631690780/LConn3 -- Line -1573549862/RConn3 -- Line -248472701/LConn3
  трансформатор КТП-631/LConn1 -- Line -248472701/RConn1
  трансформатор КТП-631/LConn2 -- Line -248472701/RConn2
  трансформатор КТП-631/LConn3 -- Line -248472701/RConn3
  Line 5eaa682b-c0d1-4c29-ad0a-d3eb85026fa4/LConn1 -- Line -993331/RConn1 -- Line -1573549862/LConn1
  Line 5eaa682b-c0d1-4c29-ad0a-d3eb85026fa4/LConn2 -- Line -993331/RConn2 -- Line -1573549862/LConn2
  Line 5eaa682b-c0d1-4c29-ad0a-d3eb85026fa4/LConn3 -- Line -993331/RConn3 -- Line -1573549862/LConn3
  трансформатор ТП-634/LConn1 -- Line 121b61d0-b677-497c-8a2a-d4a5cdbd5048/RConn1
  трансформатор ТП-634/LConn2 -- Line 121b61d0-b677-497c-8a2a-d4a5cdbd5048/RConn2
  трансформатор ТП-634/LConn3 -- Line 121b61d0-b677-497c-8a2a-d4a5cdbd5048/RConn3
  Line 74418cf8-5b73-4043-b812-f8da871132a1/LConn1 -- Line 1505548179/RConn1 -- Line 1786770246/LConn1
  Line 74418cf8-5b73-4043-b812-f8da871132a1/LConn2 -- Line 1505548179/RConn2 -- Line 1786770246/LConn2
  Line 74418cf8-5b73-4043-b812-f8da871132a1/LConn3 -- Line 1505548179/RConn3 -- Line 1786770246/LConn3
  Line 1851219918/LConn1 -- Line 1631690780/RConn1 -- Line -1382640622/LConn1
  Line 1851219918/LConn2 -- Line 1631690780/RConn2 -- Line -1382640622/LConn2
  Line 1851219918/LConn3 -- Line 1631690780/RConn3 -- Line -1382640622/LConn3
  трансформатор КТП-432/LConn1 -- Line 1786770246/RConn1
  трансформатор КТП-432/LConn2 -- Line 1786770246/RConn2
  трансформатор КТП-432/LConn3 -- Line 1786770246/RConn3
  трансформатор ТП-429/LConn1 -- Line 1851219918/RConn1
  трансформатор ТП-429/LConn2 -- Line 1851219918/RConn2
  трансформатор ТП-429/LConn3 -- Line 1851219918/RConn3
  трансформатор ТП-433/LConn1 -- Line 1921878408/RConn1
  трансформатор ТП-433/LConn2 -- Line 1921878408/RConn2
  трансформатор ТП-433/LConn3 -- Line 1921878408/RConn3
  трансформатор Т_ЗТП-1133/LConn1 -- Line 5eaa682b-c0d1-4c29-ad0a-d3eb85026fa4/RConn1
  трансформатор Т_ЗТП-1133/LConn2 -- Line 5eaa682b-c0d1-4c29-ad0a-d3eb85026fa4/RConn2
  трансформатор Т_ЗТП-1133/LConn3 -- Line 5eaa682b-c0d1-4c29-ad0a-d3eb85026fa4/RConn3
  ef7e6e5c-d6d3-47ac-94d4-f78d13d75cf1/LConn1 -- Line 74418cf8-5b73-4043-b812-f8da871132a1/RConn1
  ef7e6e5c-d6d3-47ac-94d4-f78d13d75cf1/LConn2 -- Line 74418cf8-5b73-4043-b812-f8da871132a1/RConn2
  ef7e6e5c-d6d3-47ac-94d4-f78d13d75cf1/LConn3 -- Line 74418cf8-5b73-4043-b812-f8da871132a1/RConn3
  Line 1921878408/LConn1 -- Line 815418743/RConn1 -- Line 1505548179/LConn1
  Line 1921878408/LConn2 -- Line 815418743/RConn2 -- Line 1505548179/LConn2
  Line 1921878408/LConn3 -- Line 815418743/RConn3 -- Line 1505548179/LConn3
  Source PC1_TT2/RConn1 -- fd61661e-6807-4638-8719-010892064a70/LConn1
  Source PC1_TT2/RConn2 -- fd61661e-6807-4638-8719-010892064a70/LConn2
  Source PC1_TT2/RConn3 -- fd61661e-6807-4638-8719-010892064a70/LConn3
  Line -993331/LConn1 -- fd61661e-6807-4638-8719-010892064a70/RConn1
  Line -993331/LConn2 -- fd61661e-6807-4638-8719-010892064a70/RConn2
  Line -993331/LConn3 -- fd61661e-6807-4638-8719-010892064a70/RConn3
